simulink model "equation_system_model"  (R2024a)
settings: Solver=VariableStepAuto  StartTime=0.0  StopTime=10.0  RelTol=1e-3
settings Model: Creator=andrey  LastModifiedBy=andrey

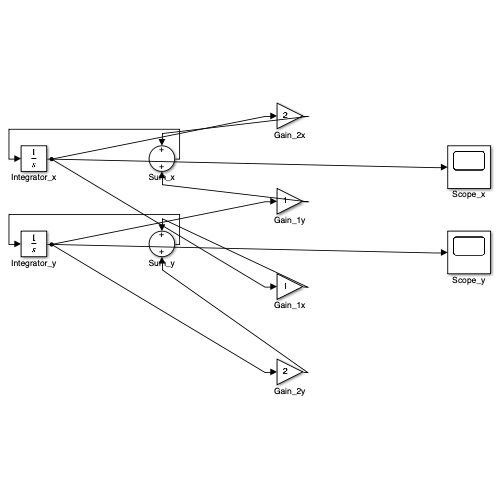
[thumbnail: Simulink's stored preview of the top-level diagram]
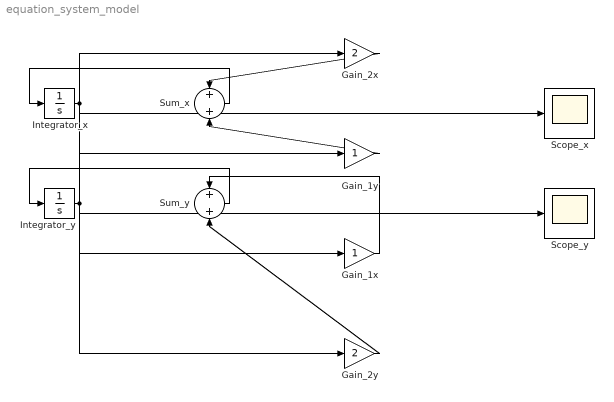
== system equation_system_model ==
  Gain_1x : Gain
  Gain_1y : Gain
  Gain_2x : Gain  Gain=2
  Gain_2y : Gain  Gain=2
  Integrator_x : Integrator  InitialCondition=-1
  Integrator_y : Integrator
  Scope_x : Scope
  Scope_y : Scope
  Sum_x : Sum
  Sum_y : Sum
  wires:
  Integrator_x/1 -> Gain_2x/1, Gain_1x/1, Scope_x/1
  Integrator_y/1 -> Gain_1y/1, Gain_2y/1, Scope_y/1
  Gain_2x/1 -> Sum_x/1
  Gain_1y/1 -> Sum_x/2
  Sum_x/1 -> Integrator_x/1
  Gain_1x/1 -> Sum_y/1
  Gain_2y/1 -> Sum_y/2
  Sum_y/1 -> Integrator_y/1
